simulink model "LKAS_AutoSave_20220216_1647"  (R2018b)
settings: Solver=FixedStepDiscrete  StartTime=0.0  StopTime=10.0  FixedStep=0.01  RelTol=1e-3
InitFcn:
  | tmpVer = ver('MATLAB');
  | tmpVer = str2num(tmpVer.Version);
  | % -------------------------------------------------------------------
  | %  MATLAB file generated by Simulink.saveVars on 21-Nov-2019 10:06:14
  | %  MATLAB version: 7.13.0.564 (R2011b)
  | % -------------------------------------------------------------------
  | 
  | 
  | SInt16 = Simulink.AliasType;
  | SInt16.Description = 'Num';
  | if (tmpVer > 7.11)
  | 	SInt16.DataScope = 'Auto';
  | end
  | SInt16.HeaderFile = 'Rte_Type.h';
  | SInt16.BaseType = 'int16';
  | 
  | SInt32 = Simulink.AliasType;
  | SInt32.Description = 'Num';
  | if (tmpVer > 7.11)
  | 	SInt32.DataScope = 'Auto';
  | end
  | SInt32.HeaderFile = 'Rte_Type.h';
  | SInt32.BaseType = 'int32';
  | 
  | SInt8 = Simulink.AliasType;
  | SInt8.Description = 'Num';
  | if (tmpVer > 7.11)
  | 	SInt8.DataScope = 'Auto';
  | end
  | SInt8.HeaderFile = 'Rte_Type.h';
  | SInt8.BaseType = 'int8';
  | 
  | T_A_m2_1024_1_u32 = Simulink.NumericType;
  | T_A_m2_1024_1_u32.Description = 'm2 (square meters  (m2))';
  | if (tmpVer > 7.11)
  | 	T_A_m2_1024_1_u32.DataScope = 'Auto';
  | end
  | T_A_m2_1024_1_u32.HeaderFile = 'Rte_Type.h';
  | T_A_m2_1024_1_u32.DataTypeMode = 'Fixed-point: slope and bias scaling';
  | T_A_m2_1024_1_u32.SignednessBool = false;
  | T_A_m2_1024_1_u32.WordLength = 32;
  | T_A_m2_1024_1_u32.FixedExponent = -10;
  | T_A_m2_1024_1_u32.SlopeAdjustmentFactor = 1;
  | T_A_m2_1024_1_u32.Bias = 0;
  | T_A_m2_1024_1_u32.DataTypeOverride = 'Inherit';
  | T_A_m2_1024_1_u32.IsAlias = true;
  | 
  | T_A_m2_65536_1_u16 = Simulink.NumericType;
  | T_A_m2_65536_1_u16.Description = 'm2 (square meters  (m2))';
  | if (tmpVer > 7.11)
  | 	T_A_m2_65536_1_u16.DataScope = 'Auto';
  | end
  | T_A_m2_65536_1_u16.HeaderFile = 'Rte_Type.h';
  | T_A_m2_65536_1_u16.DataTypeMode = 'Fixed-point: slope and bias scaling';
  | T_A_m2_65536_1_u16.SignednessBool = false;
  | T_A_m2_65536_1_u16.WordLength = 16;
  | T_A_m2_65536_1_u16.FixedExponent = -16;
  | T_A_m2_65536_1_u16.SlopeAdjustmentFactor = 1;
  | T_A_m2_65536_1_u16.Bias = 0;
  | T_A_m2_65536_1_u16.DataTypeOverride = 'Inherit';
  | ... (+4647 lines)
StopFcn:
  | clear  T_A_m2_1024_1_u32 T_A_m2_65536_1_u16 T_A_m2_Float32 T_A_mm2_10_1_u16 T_A_mm2_4_1_s16 T_A_mm2_Float32 T_Cnt_Num_10_1_u32 T_Cnt_Num_1_1_s16 T_Cnt_Num_1_1_s32 T_Cnt_Num_1_1_s8 T_Cnt_Num_1_1_u16 T_Cnt_Num_1_1_u32 T_Cnt_Num_1_1_u8 T_E_J_1_1_s32 T_E_J_Float32 T_E_kJ_128_1_s32 T_E_kJ_Float32 T_E_kwh_10_1_u16 T_E_kwh_Float32 T_Epl_kwhpkm_100_1_u16 T_Epl_kwhpkm_Float32 T_F_N_1_1_s16 T_F_N_Float32 T_I_A_1000_1_u16 T_I_A_1048576_1_s32 T_I_A_2048_1_s16 T_I_A_32_1_s16 T_I_A_Float32 T_I_mA_1_1_s16 T_I_mA_32768_128_s16 T_I_mA_Float32 T_J_kgpm2_128_1_u16 T_J_kgpm2_Float32 T_K_NA_1000_1_s16 T_K_NA_100_1_s16 T_K_NA_100_1_u16 T_K_NA_1024_1_s16 T_K_NA_1024_1_u16 T_K_NA_128_1_s16 T_K_NA_128_1_u16 T_K_NA_128_1_u8 T_K_NA_16777216_1_u32 T_K_NA_16_1_s16 T_K_NA_16_1_u16 T_K_NA_16_1_u8 T_K_NA_1_16_u16 T_K_NA_1_1_s16 T_K_NA_1_1_u16 T_K_NA_1_1_u8 T_K_NA_32768_1_s16 T_K_NA_32768_1_u16 T_K_NA_32_1_s8 T_K_NA_4096_1_u16 T_K_NA_4194304_1_s32 T_K_NA_4194304_1_u16 T_K_NA_65536_1_s32 T_K_NA_65536_1_u16 T_K_NA_8192_1_s16 T_K_NA_8_1_s16 T_K_NA_Float32 T_M_Nm_16_1_s16 T_M_Nm_1_1_s16 T_M_Nm_32768_1_s16 T_M_Nm_32_1_s16 T_M_Nm_4_1_s16 T_M_Nm_512_1_s16 T_M_Nm_Float32 T_P_W_1_4_s16 T_P_W_1_8_s16 T_P_W_Float32 T_P_kW_128_1_s16 T_P_kW_1_8_s16 T_P_kW_8_1_s32 T_P_kW_Float32 T_Pct_pct_1024_1_s32 T_Pct_pct_1024_1_u32 T_Pct_pct_10_1_s16 T_Pct_pct_10_1_u32 T_Pct_pct_128_100_s8 T_Pct_pct_1_1_s16 T_Pct_pct_1_4_u8 T_Pct_pct_255_100_u16 T_Pct_pct_255_100_u8 T_Pct_pct_256_1_s16 T_Pct_pct_256_1_u16 T_Pct_pct_65535_100_u16 T_Pct_pct_Float32 T_R_ohm_1024_1_s16 T_R_ohm_32_1_s16 T_R_ohm_Float32 T_TK_K_16_1_s16 T_TK_K_Float32 T_T_degC_10_400_1_u16 T_T_degC_16_1_s16 T_T_degC_1_40_1_u8 T_T_degC_2_80_1_u8 T_T_degC_Float32 T_U_V_1000_1_u16 T_U_V_10_1_u8 T_U_V_200_1_u8 T_U_V_32_1_s16 T_U_V_4096_1_s16 T_U_V_512_1_s16 T_U_V_65535_8_u16 T_U_V_8192_1_u16 T_U_V_Float32 T_U_mV_1_1_s16 T_U_mV_256_20_u16 T_U_mV_Float32 T_V_l_256_1_s16 T_V_l_4096_1_s16 T_V_l_64_1_s16 T_V_l_65535_100_u16 T_V_l_Float32 T_V_ml_128_1_s16 T_V_ml_1_1_s16 T_V_ml_32768_1_s16 T_V_ml_Float32 T_V_ul_32_1_u16 T_V_ul_Float32 T_Vpl_clpkm_512_1_u16 T_Vpl_clpkm_Float32 T_a_kphps_16_1_s16 T_a_kphps_Float32 T_a_mps2_128_1_s16 T_a_mps2_Float32 T_c_MJpkg_256_1_s16 T_c_MJpkg_Float32 T_c_kJpgpK_1024_1_s16 T_c_kJpgpK_Float32 T_c_kJpkgpK_128_1_u16 T_c_kJpkgpK_Float32 T_chrg_Ah_1_1_s16 T_chrg_Ah_1_1_u16 T_chrg_Ah_1_1_u8 T_chrg_Ah_256_1_u16 T_chrg_Ah_4194304_1_s32 T_chrg_Ah_512_1_u16 T_chrg_Ah_8_1_u16 T_chrg_Ah_Float32 T_cmp_NA_100_1_s16 T_cmp_NA_128_1_s16 T_cmp_NA_16_1_s16 T_cmp_NA_32768_1_u16 T_cmp_NA_Float32 T_d2n_rpmps2_4_1_s16 T_d2n_rpmps2_Float32 T_dPct_pctps_16_1_s16 T_dPct_pctps_256_1_s16 T_dPct_pctps_Float32 T_dT_degCps_128_1_s16 T_dT_degCps_Float32 T_dV_lph_1_1_s16 T_dV_lph_Float32 T_dV_lpm_128_1_s16 T_dV_lpm_32_1_s16 T_dV_lpm_Float32 T_dV_lps_1024_1_u16 T_dV_lps_4_1_u16 T_dV_lps_Float32 T_dV_mlps_1024_1_s16 T_dV_mlps_Float32 T_d_BitField16 T_dm_gps_128_1_s16 T_dm_gps_128_1_u16 T_dm_gps_256_1_u16 T_dm_gps_Float32 T_dm_mgps_1_1_s16 T_dm_mgps_Float32 T_dn_rpmps_1_1_s16 T_dn_rpmps_2_1_s16 T_dn_rpmps_Float32 T_dp_Paps_1_1_s16 T_dp_Paps_Float32 T_dp_kPaps_1_1_s16 T_dp_kPaps_8_1_s16 T_dp_kPaps_Float32 T_dphi_degps_128_1_s16 T_dphi_degps_8_1_s16 T_dphi_degps_Float32 T_dr_ps_256_1_s16 T_dr_ps_Float32 T_drho_mgplps_1_2_s16 T_drho_mgplps_Float32 T_e_NA_1_1_u8 T_f_Hz_1_1_u16 T_f_Hz_1_1_u32 T_f_Hz_64_1_u16 T_f_Hz_8_1_s16 T_f_Hz_Float32 T_g_BitField32 T_l_km_16_1_s16 T_l_km_1_1_u16 T_l_km_1_1_u32 T_l_km_Float32 T_l_m_1024_1_s16 T_l_m_16_1_s16 T_l_m_1_1_u32 T_l_m_Float32 T_l_mm_16_1_s16 T_l_mm_1_1_u16 T_l_mm_4096_1_s16 T_l_mm_4_1_u8 T_l_mm_64_1_s16 T_l_mm_Float32 T_m_g_1_1_s16 T_m_g_2048_1_s16 T_m_g_32_1_u16 T_m_g_Float32 T_m_kg_1024_1_s16 T_m_kg_1_1_s16 T_m_kg_1_1_u32 T_m_kg_Float32 T_m_mg_128_1_s16 T_m_mg_32_1_s16 T_m_mg_Float32 T_n_rpm_1_1_s16 T_n_rpm_1_25_u8 T_n_rpm_256_50_u16 T_n_rpm_2_25_u8 T_n_rpm_4_1_u16 T_n_rpm_Float32 T_p_MPa_64_1_s16 T_p_MPa_Float32 T_p_Pa_1_1_s16 T_p_Pa_Float32 T_p_kPa_1_10_u16 T_p_kPa_1_1_s16 T_p_kPa_1_1_u8 T_p_kPa_256_1_u16 T_p_kPa_32_1_u16 T_p_kPa_64_1_s16 T_p_kPa_Float32 T_phi_deg_100_1_s16 T_phi_deg_1024_1_s16 T_phi_deg_128_1_s16 T_phi_deg_1_1_u8 T_phi_deg_256_1_s16 T_phi_deg_2_1_s8 T_phi_deg_32_1_s16 T_phi_deg_512_6_s32 T_phi_deg_Float32 T_phi_rad_2048_1_s16 T_phi_rad_Float32 T_r_NA_1024_1_s16 T_r_NA_1024_1_u16 T_r_NA_16384_1_s16 T_r_NA_16_1_s16 T_r_NA_256_1_s8 T_r_NA_256_1_u16 T_r_NA_32768_1_u16 T_r_NA_32_1_u16 T_r_NA_4096_1_s16 T_r_NA_65535_2_u16 T_r_NA_8192_1_u16 T_r_NA_Float32 T_rho_gpl_8192_1_s16 T_rho_gpl_Float32 T_rho_kgpm3_16_1_s16 T_rho_kgpm3_Float32 T_rho_mgpl_1_1_s16 T_rho_mgpl_64_1_s16 T_rho_mgpl_Float32 T_t_hour_1_1_s16 T_t_hour_Float32 T_t_m_1_1_u16 T_t_m_Float32 T_t_ms_1_1_s16 T_t_ms_1_1_u16 T_t_ms_1_1_u32 T_t_ms_4096_1_s16 T_t_ms_64_1_s16 T_t_ms_Float32 T_t_s_1000_1_s16 T_t_s_100_1_s16 T_t_s_10_1_s16 T_t_s_10_1_u16 T_t_s_1_1_s16 T_t_s_1_1_u16 T_t_s_1_1_u32 T_t_s_Float32 T_t_us_10_1_u32 T_t_us_1_1_s16 T_t_us_1_1_u32 T_t_us_1_4_u16 T_t_us_Float32 T_v_kph_1_1_u8 T_v_kph_64_1_s16 T_v_kph_64_1_u16 T_v_kph_Float32 T_v_mps_256_1_s16 T_v_mps_Float32 T_w_radps_32_1_s16 T_w_radps_Float32 T_y_BitField8 T_y_BitFieldDiagProgress T_y_BitFieldDiagStatus T_y_NA_1_1_u8 SInt16 SInt32 SInt8 T_BOOLEAN UInt16 UInt32 UInt8 s16 s32 s8 u16 u32 u8
model workspace (MAT data in the model file):
  MCOS : class17 (value not decoded)
  MCOS : class17 (value not decoded)
  MCOS : class17 (value not decoded)
  MCOS : class17 (value not decoded)
  MCOS : class17 (value not decoded)
  MCOS : class17 (value not decoded)
  MCOS : class17 (value not decoded)
  MCOS : class17 (value not decoded)
  MCOS : class17 (value not decoded)
  MCOS : class17 (value not decoded)
  MCOS : class17 (value not decoded)
  MCOS : class17 (value not decoded)
  MCOS : class17 (value not decoded)
  MCOS : class17 (value not decoded)
  MCOS : class17 (value not decoded)
  MCOS : class17 (value not decoded)
  MCOS : class17 (value not decoded)
  MCOS : class17 (value not decoded)
  MCOS : class17 (value not decoded)
  MCOS : class17 (value not decoded)
  MCOS : class17 (value not decoded)
  MCOS : class17 (value not decoded)
  MCOS : class17 (value not decoded)
  MCOS : class17 (value not decoded)
  MCOS : class17 (value not decoded)
  MCOS : class17 (value not decoded)
  MCOS : class17 (value not decoded)
  MCOS : class17 (value not decoded)
  MCOS : class17 (value not decoded)
  MCOS : class17 (value not decoded)
  MCOS : class17 (value not decoded)
  MCOS : class17 (value not decoded)
  MCOS : class17 (value not decoded)
  MCOS : class17 (value not decoded)
  MCOS : class17 (value not decoded)
  MCOS : class17 (value not decoded)
  MCOS : class17 (value not decoded)
  MCOS : class17 (value not decoded)
  MCOS : class17 (value not decoded)
  MCOS : class17 (value not decoded)
  MCOS : class17 (value not decoded)
  MCOS : class17 (value not decoded)
  MCOS : class17 (value not decoded)
  MCOS : class17 (value not decoded)
  MCOS : class17 (value not decoded)
  MCOS : class17 (value not decoded)
  MCOS : class17 (value not decoded)
  MCOS : class17 (value not decoded)
  MCOS : class17 (value not decoded)
  MCOS : class17 (value not decoded)
  MCOS : class17 (value not decoded)
  MCOS : class17 (value not decoded)
  MCOS : class17 (value not decoded)
  MCOS : class17 (value not decoded)
  MCOS : class17 (value not decoded)
  MCOS : class17 (value not decoded)
  MCOS : class17 (value not decoded)
  MCOS : class17 (value not decoded)
  MCOS : class17 (value not decoded)
  MCOS : class17 (value not decoded)
  MCOS : class17 (value not decoded)
  MCOS : class17 (value not decoded)
  MCOS : class17 (value not decoded)
  MCOS : class17 (value not decoded)
  MCOS : class17 (value not decoded)
  MCOS : class17 (value not decoded)
  MCOS : class17 (value not decoded)
  MCOS : class17 (value not decoded)
  MCOS : class17 (value not decoded)
  MCOS : class17 (value not decoded)
  MCOS : class17 (value not decoded)
  MCOS : class17 (value not decoded)
  MCOS : class17 (value not decoded)
  MCOS : class17 (value not decoded)
  MCOS : class17 (value not decoded)
  MCOS : class17 (value not decoded)
  MCOS : class17 (value not decoded)
  MCOS : class17 (value not decoded)
  MCOS : class17 (value not decoded)
  MCOS : class17 (value not decoded)
  MCOS : class17 (value not decoded)
  MCOS : class17 (value not decoded)
  MCOS : class17 (value not decoded)
  MCOS : class17 (value not decoded)
  MCOS : class17 (value not decoded)
  MCOS : class17 (value not decoded)
  MCOS : class17 (value not decoded)
  MCOS : class17 (value not decoded)
  MCOS : class17 (value not decoded)
  MCOS : class17 (value not decoded)
  MCOS : class17 (value not decoded)
  MCOS : class17 (value not decoded)
  MCOS : class17 (value not decoded)
  MCOS : class17 (value not decoded)
  MCOS : class17 (value not decoded)
  MCOS : class17 (value not decoded)
  MCOS : class17 (value not decoded)
  MCOS : class17 (value not decoded)
  MCOS : class17 (value not decoded)
  MCOS : class17 (value not decoded)
  MCOS : class17 (value not decoded)
  MCOS : class17 (value not decoded)
undefined symbols (not defined in the file): LKA_CarWidth, LKA_SampleTime, LKA_StrRatio_C, LKA_Veh2CamL_C, LKA_Veh2CamW_C, LKA_WhlBaseL_C, LL_CompHdAg_C, LL_CompSWA_C, LL_CrvtPrvwT_C, LL_DesDvt_C, LL_DvtComp_C, LL_DvtPrvwT_C, LL_DvtSpdDet_vDvtSpdMin_C, LL_HandsOff_ExitTime, LL_HandsOff_TextTime, LL_HandsOff_WarnTime, LL_HdAgExT_C, LL_HdAgPrvwT_C, LL_LAccMax_C, LL_LAccRMax_C, LL_LDW_EarliestWarnLine_C, LL_LDW_LatestWarnLine_C, LL_LDWS_SUPPRESS_HEADING, LL_LFClb_TFC_FfCtlRatio_C, LL_LFClb_TFC_KdBalance_C, LL_LFClb_TFC_KdMaxSWA_C, LL_LFClb_TFC_KdV1_C, LL_LFClb_TFC_KdV2_C, LL_LFClb_TFC_KdVehSpdLwr_C, LL_LFClb_TFC_KdVehSpdUpr_C, LL_LFClb_TFC_Ki_C, LL_LFClb_TFC_KiMaxSWA_C, LL_LFClb_TFC_Kp_C, LL_LFClb_TFC_KpKlat_C, LL_LFClb_TFC_KpV1_C, LL_LFClb_TFC_KpV2_C, LL_LFClb_TFC_KpVehSpdLwr_C, LL_LFClb_TFC_KpVehSpdUpr_C, LL_LFClb_TFC_PrvwT_C, LL_LKA_EarliestWarnLine_C, LL_LKA_LatestWarnLine_C, LL_LKAExPrcs_ExitC0Dvt, LL_LKAExPrcs_ExitC0Swt, LL_LKAExPrcs_tiExitTime1, LL_LKAExPrcs_tiExitTime2, LL_LKAExPrcs_tiExitTime3, LL_LKAS_OUT_OF_CONTROL_LAT_VEL, LL_LKAS_OUT_OF_CONTROL_TTLC, LL_LKASWASyn_M0, LL_LKASWASyn_M1, LL_LKASWASyn_M2, LL_LKASWASyn_M3K, LL_LKASWASyn_SWAaddMax, LL_LKASWASyn_T2, LL_LKASWASyn_tiTrqSwaRtTime, LL_LKASWASyn_tiTrqSwaTime, LL_LKASWASyn_TrqMax, LL_LKASWASyn_TrqSwaAddSwt, LL_LKASWASyn_TrqSwaRateDiff, LL_LSpdCompT_C ... (+43)
libraries: simulink x136, canmsglib x8, dspstat3 x3, simulink_extras x1
(part 16 of 20)

== system LKAS_AutoSave_20220216_1647/LKAS/LL/LLOn/LL State Determination (LLStateDet)/LL State Machine Conditions (LLSMCon)/Disable Condition (DisblC)/Driver Intent Condition (DrvInttC)/Driver Action Detection (DrvActnDet) ==
  DrvActnDet_phiSWA : Inport
  DrvActnDet_dphiSWA_Speed : Inport  Port=2
  DrvActnDet_aLAcc : Inport  Port=3
  DrvActnDet_aFAcc : Inport  Port=4
  DrvActnDet_bsEPSInfo : Inport  Port=5
  DrvInttC_bsLLClb : Inport  Port=6
  Abs2 : Abs  OutDataTypeStr=single
  Abs3 : Abs  OutDataTypeStr=single
  Abs4 : Abs  OutDataTypeStr=single
  Bus Creator : BusCreator  Inputs=4
  Bus Selector : BusSelector  OutputSignals=EPS_LKA_State
  Bus Selector1 : BusSelector  OutputSignals=bsLLSMConClb.DisblCClb.LL_MAX_STEER_ANGLE_DISABLE,bsLLSMConClb.DisblCClb.LL_MAX_STEER_SPEED_DISABLE,bsLLSMConClb.DisblCClb.LL_MAX_LAT_ACC_DISABLE,bsLLSMConClb.DisblCClb.LL_MAX_LONG_ACC_DISABLE,bsLLSMConClb.DisblCClb.LL_MAX_LONG_DECEL_DISABLE
  Compare To Constant : simulink/Logic and Bit Operations/Compare To Constant  relop=~=  const=3.0  OutDataTypeStr=boolean
  Compare To Constant2 : simulink/Logic and Bit Operations/Compare To Constant  relop===  const=0  OutDataTypeStr=boolean
  Interval Test Dynamic : simulink/Logic and Bit Operations/Interval Test Dynamic  IntervalClosedRight=off  IntervalClosedLeft=off  OutDataTypeStr=boolean
      settings: SourceProductName=Simulink  SourceProductBaseCode=SL
  Logical Operator : Logic  Operator=OR  Inputs=4  AllPortsSameDT=off  OutDataTypeStr=boolean
  Logical Operator1 : Logic  AllPortsSameDT=off  OutDataTypeStr=boolean
  Relational Operator1 : RelationalOperator  OutDataTypeStr=boolean  RndMeth=Nearest
  Relational Operator2 : RelationalOperator  OutDataTypeStr=boolean  RndMeth=Nearest
  Relational Operator3 : RelationalOperator  OutDataTypeStr=boolean  RndMeth=Nearest
  Unary Minus : UnaryMinus
  DrvActnDet_stTkOvStActvFlg : Outport
  DrvActnDet : Outport  Port=2
  wires:
  Abs2/1 -> Relational Operator1/1
  Bus Selector1/1 -> Relational Operator1/2  "<LL_MAX_STEER_ANGLE_DISABLE>"
  Abs3/1 -> Relational Operator2/1
  Bus Selector1/2 -> Relational Operator2/2  "<LL_MAX_STEER_SPEED_DISABLE>"
  DrvActnDet_phiSWA/1 -> Abs2/1
  DrvActnDet_aLAcc/1 -> Abs4/1
  Abs4/1 -> Relational Operator3/1
  Bus Selector1/3 -> Relational Operator3/2  "<LL_MAX_LAT_ACC_DISABLE>"
  Bus Selector1/5 -> Unary Minus/1  "<LL_MAX_LONG_DECEL_DISABLE>"
  DrvActnDet_aFAcc/1 -> Interval Test Dynamic/2
  Interval Test Dynamic/1 -> Compare To Constant2/1
  Bus Selector1/4 -> Interval Test Dynamic/1  "<LL_MAX_LONG_ACC_DISABLE>"
  Unary Minus/1 -> Interval Test Dynamic/3
  Relational Operator3/1 -> Logical Operator1/1
  DrvActnDet_bsEPSInfo/1 -> Bus Selector/1
  Bus Selector/1 -> Compare To Constant/1  "<EPS_LKA_State>"
  Compare To Constant/1 -> Logical Operator1/2
  Logical Operator/1 -> DrvActnDet_stTkOvStActvFlg/1
  Relational Operator1/1 -> Bus Creator/1, Logical Operator/1  "phiSWA_Thres"
  Bus Creator/1 -> DrvActnDet/1
  Compare To Constant2/1 -> Bus Creator/4, Logical Operator/4  "aFLAcc_Thres"
  Logical Operator1/1 -> Bus Creator/3, Logical Operator/3  "aLAcc_Thres"
  Relational Operator2/1 -> Bus Creator/2, Logical Operator/2  "dphiSWARate_Thres"
  DrvActnDet_dphiSWA_Speed/1 -> Abs3/1
  DrvInttC_bsLLClb/1 -> Bus Selector1/1

== system LKAS_AutoSave_20220216_1647/LKAS/LL/LLOn/LL State Determination (LLStateDet)/LL State Machine Conditions (LLSMCon)/Disable Condition (DisblC)/Driver Intent Condition (DrvInttC)/Driver Release Detection (DrvRlsDet) ==
  DrvRlsDet_bsEPSInfo : Inport
  DrvRlsDet_bsLLClb : Inport  Port=2
  Abs : Abs
  Bus Selector2 : BusSelector  OutputSignals=EPS_LKA_State,EPS_SW_Trq
  Bus Selector3 : BusSelector  OutputSignals=bsLLSMConClb.DisblCClb.LL_RlsDet_tiTrqChkT_DISABLE,bsLLSMConClb.DisblCClb.LL_RlsDet_tiTrqChkT_EPS_DISABLE,bsConstantClb.LKA_SampleTime,bsLLSMConClb.DisblCClb.LL_HandsOff_ExitTime
  Compare1 : simulink/Logic and Bit Operations/Compare To Constant  relop===  const=3  OutDataTypeStr=boolean
  Compare3 : simulink/Logic and Bit Operations/Compare To Constant  relop===  const=3  OutDataTypeStr=boolean
  Compare4 : simulink/Logic and Bit Operations/Compare To Constant  relop===  const=1  OutDataTypeStr=boolean
  Divide : Product  Inputs=**
  ExitCount : Subsystem
  Logical Operator1 : Logic  AllPortsSameDT=off  OutDataTypeStr=boolean
  Logical Operator2 : Logic  Operator=OR  AllPortsSameDT=off  OutDataTypeStr=boolean
  Relational Operator : RelationalOperator  Operator=<=  OutDataTypeStr=boolean  RndMeth=Nearest
  Switch : Switch  Criteria=u2 > Threshold
  DrvRlsDet_stDrvRlsDetFlg : Outport
  wires:
  Logical Operator1/1 -> Divide/1
  DrvRlsDet_bsEPSInfo/1 -> Bus Selector2/1
  Bus Selector2/1 -> Compare1/1, Compare4/1, Compare3/1  "<EPS_LKA_State>"
  Bus Selector2/2 -> Abs/1  "<EPS_SW_Trq>"
  Relational Operator/1 -> ExitCount/Enable, Logical Operator1/2
  Compare1/1 -> Switch/2
  Compare3/1 -> Logical Operator2/2
  Bus Selector3/2 -> Switch/1  "<LL_RlsDet_tiTrqChkT_EPS_DISABLE>"
  Switch/1 -> Relational Operator/2
  Logical Operator2/1 -> Logical Operator1/1
  Compare4/1 -> Logical Operator2/1
  Abs/1 -> Relational Operator/1
  DrvRlsDet_bsLLClb/1 -> Bus Selector3/1
  Bus Selector3/1 -> Switch/3  "<LL_RlsDet_tiTrqChkT_DISABLE>"
  Bus Selector3/3 -> Divide/2  "<LKA_SampleTime>"
  Bus Selector3/4 -> ExitCount/2(ExitTime)  "<LL_HandsOff_ExitTime>"
  ExitCount/1(Out) -> DrvRlsDet_stDrvRlsDetFlg/1
  Divide/1 -> ExitCount/1(SampleTime)

== system LKAS_AutoSave_20220216_1647/LKAS/LL/LLOn/LL State Determination (LLStateDet)/LL State Machine Conditions (LLSMCon)/Disable Condition (DisblC)/Driver Intent Condition (DrvInttC)/Take-Over Steering Check (TkOvStChk) ==
  TkOvStChk_bsEPSInfo : Inport
  TkOvStChk_bsLLClb : Inport  Port=2
  TkOvStChk_bsVehSpd : Inport  Port=3
  TkOvStChk_crPrvwCrvt : Inport  Port=4
  Abs : Abs
  Bus Selector : BusSelector  OutputSignals=EPS_SW_Trq
  Bus Selector1 : BusSelector  OutputSignals=bsLLSMConClb.DisblCClb.LL_MAX_DRIVER_TORQUE_DISABLE,bsLLSMConClb.DisblCClb.LL_TkOvStChk_tiTrqChkT,bsLLSMConClb.DisblCClb.LL_TkOvStChk_tiTDelTime,bsConstantClb.LKA_SampleTime
  MATLAB Function : MATLAB Function  TreatAsAtomicUnit=on
  Saturation : Saturate  UpperLimit=80  LowerLimit=60
      settings: AttributesFormatString="Min = %<LowerLimit>  Max = %<UpperLimit>"
  Sum Condition1 : Subsystem  TreatAsAtomicUnit=on
  Time Delay (TDel) : Subsystem
  TkOvStChk_stTkOvStChk : Outport
  wires:
  Sum Condition1/1(Out) -> Time Delay (TDel)/1(TDel_stFlgIn)
  Saturation/1 -> MATLAB Function/1(VehSpd)
  TkOvStChk_bsEPSInfo/1 -> Bus Selector/1
  Bus Selector/1 -> Abs/1  "<EPS_SW_Trq>"
  Abs/1 -> MATLAB Function/2(EPSTrq)
  Bus Selector1/1 -> MATLAB Function/3(DisableTrq)  "<LL_MAX_DRIVER_TORQUE_DISABLE>"
  MATLAB Function/1(stDvrTkConFlg) -> Sum Condition1/Enable
  Bus Selector1/2 -> Sum Condition1/2(Sum)  "<LL_TkOvStChk_tiTrqChkT>"
  Time Delay (TDel)/1(TDel_stFlgOut) -> TkOvStChk_stTkOvStChk/1
  TkOvStChk_bsVehSpd/1 -> Saturation/1
  Bus Selector1/3 -> Time Delay (TDel)/3(TDel_tiTDel)  "<LL_TkOvStChk_tiTDelTime>"
  Bus Selector1/4 -> Sum Condition1/1(In), Time Delay (TDel)/2(SampleTime)  "<LKA_SampleTime>"
  TkOvStChk_crPrvwCrvt/1 -> MATLAB Function/4(PrvwCrvt)
  TkOvStChk_bsLLClb/1 -> Bus Selector1/1

== system LKAS_AutoSave_20220216_1647/LKAS/LL/LLOn/LL State Determination (LLStateDet)/LL State Machine Conditions (LLSMCon)/Disable Condition (DisblC)/LDW Alarm Timeout (LDWAlrmTOut)/If Action Subsystem ==
  In : Inport
  Sum : Inport  Port=2
  Action Port : ActionPort  InitializeStates=reset
      settings: AttributesFormatString=states = %<InitializeStates>
  Add1 : Sum  OutDataTypeStr=single
  Memory : Memory  InheritSampleTime=on
  Relational Operator : RelationalOperator  OutDataTypeStr=boolean  RndMeth=Nearest
  Saturation : Saturate  UpperLimit=10  LowerLimit=0
      settings: AttributesFormatString="Min = %<LowerLimit>  Max = %<UpperLimit>"
  Out : Outport  InitialOutput=0
      settings: AttributesFormatString=%<OutputWhenDisabled> = %<InitialOutput>
  wires:
  Sum/1 -> Relational Operator/2
  In/1 -> Add1/1
  Memory/1 -> Add1/2
  Saturation/1 -> Memory/1, Relational Operator/1
  Add1/1 -> Saturation/1
  Relational Operator/1 -> Out/1

== system LKAS_AutoSave_20220216_1647/LKAS/LL/LLOn/LL State Determination (LLStateDet)/LL State Machine Conditions (LLSMCon)/Disable Condition (DisblC)/LDW Alarm Timeout (LDWAlrmTOut)/If Action Subsystem1 ==
  Action Port : ActionPort  InitializeStates=reset
      settings: AttributesFormatString=states = %<InitializeStates>
  Constant : Constant  Value=0  OutDataTypeStr=boolean
  Out1 : Outport  InitialOutput=0
      settings: AttributesFormatString=%<OutputWhenDisabled> = %<InitialOutput>
  wires:
  Constant/1 -> Out1/1

== system LKAS_AutoSave_20220216_1647/LKAS/LL/LLOn/LL State Determination (LLStateDet)/LL State Machine Conditions (LLSMCon)/Disable Condition (DisblC)/LKA Own Condition (LKAOwnC)/EPS Condition (EPSC) ==
  EPSC_tiDelT_C : Inport
  EPSC_tiLKA_SampleTime : Inport  Port=2
  EPSC_bsEPSInfo : Inport  Port=3
  EPSC_bsLLState : Inport  Port=4
  Bus Selector : BusSelector  OutputSignals=EPS_LKA_State
  Bus Selector1 : BusSelector  OutputSignals=LKA_State
  If : If  NumInputs=2  IfExpression=u2 ==3 & u1 ~=1  ElseIfExpressions=(u2 == 4 | u2 == 5)& u1 ~= 3
  If Action Subsystem : Subsystem  TreatAsAtomicUnit=on
  If Action Subsystem1 : Subsystem  TreatAsAtomicUnit=on
  If Action Subsystem3 : Subsystem  TreatAsAtomicUnit=on
  Merge : Merge  Inputs=3
  Sum Condition1 : Subsystem  TreatAsAtomicUnit=on
  EPSC_stEPSC : Outport
  wires:
  EPSC_bsEPSInfo/1 -> Bus Selector/1
  Sum Condition1/1(Out) -> EPSC_stEPSC/1
  If Action Subsystem1/1(Out) -> Merge/2
  If Action Subsystem/1(Out) -> Merge/1
  If/1 -> If Action Subsystem/Action
  If/3 -> If Action Subsystem3/Action
  If/2 -> If Action Subsystem1/Action
  If Action Subsystem3/1(Out) -> Merge/3
  Merge/1 -> Sum Condition1/Enable
  Bus Selector/1 -> If/1  "<EPS_LKA_State>"
  EPSC_bsLLState/1 -> Bus Selector1/1
  Bus Selector1/1 -> If/2  "<LKA_State>"
  EPSC_tiDelT_C/1 -> Sum Condition1/2(Sum)
  EPSC_tiLKA_SampleTime/1 -> Sum Condition1/1(SampleTime)

== system LKAS_AutoSave_20220216_1647/LKAS/LL/LLOn/LL State Determination (LLStateDet)/LL State Machine Conditions (LLSMCon)/Disable Condition (DisblC)/LKA Own Condition (LKAOwnC)/LKA Own Condition Synthesis (LKAOwnCSyn) ==
  LKAOwnCSyn_stDACMode : Inport
  LKAOwnCSyn_stVehLSpdC : Inport  Port=2
  LKAOwnCSyn_stVehPosChk : Inport  Port=3
  LKAOwnCSyn_stEPSCtlEC : Inport  Port=4
  Compare To Constant : simulink/Logic and Bit Operations/Compare To Constant  relop===  const=2  OutDataTypeStr=boolean
  Compare To Constant1 : simulink/Logic and Bit Operations/Compare To Constant  relop===  const=1  OutDataTypeStr=boolean
  Compare To Constant2 : simulink/Logic and Bit Operations/Compare To Constant  relop===  const=1  OutDataTypeStr=boolean
  Compare To Constant3 : simulink/Logic and Bit Operations/Compare To Constant  relop===  const=1  OutDataTypeStr=boolean
  Logical Operator : Logic  AllPortsSameDT=off  OutDataTypeStr=boolean
  Logical Operator1 : Logic  Operator=OR  Inputs=3  AllPortsSameDT=off  OutDataTypeStr=boolean
  LKAOwnCSyn_stLKAOwnCSyn : Outport
  wires:
  LKAOwnCSyn_stDACMode/1 -> Compare To Constant/1
  LKAOwnCSyn_stVehPosChk/1 -> Compare To Constant1/1
  Logical Operator/1 -> LKAOwnCSyn_stLKAOwnCSyn/1
  LKAOwnCSyn_stEPSCtlEC/1 -> Compare To Constant2/1
  Compare To Constant2/1 -> ?
  Compare To Constant1/1 -> Logical Operator1/2
  Compare To Constant/1 -> Logical Operator/1
  Logical Operator1/1 -> Logical Operator/2
  LKAOwnCSyn_stVehLSpdC/1 -> Compare To Constant3/1
  Compare To Constant3/1 -> Logical Operator1/1

== system LKAS_AutoSave_20220216_1647/LKAS/LL/LLOn/LL State Determination (LLStateDet)/LL State Machine Conditions (LLSMCon)/Disable Condition (DisblC)/LKA Own Condition (LKAOwnC)/Vehicle Lateral Speed Condition (VehLSpdC) ==
  VehLSpdC_bsTTLC : Inport
  VehLSpdC_vVehLSpdMax_C : Inport  Port=2
  Abs : Abs
  Abs1 : Abs
  Bus Selector : BusSelector  OutputSignals=vLft,vRgt
  Logical Operator : Logic  Operator=OR  AllPortsSameDT=off  OutDataTypeStr=boolean
  Relational Operator1 : RelationalOperator  OutDataTypeStr=boolean  RndMeth=Nearest
  Relational Operator2 : RelationalOperator  OutDataTypeStr=boolean  RndMeth=Nearest
  VehLSpdC_stVehLSpdC : Outport
  wires:
  VehLSpdC_bsTTLC/1 -> Bus Selector/1
  Abs/1 -> Relational Operator1/1
  Bus Selector/1 -> Abs/1  "<vLft>"
  Bus Selector/2 -> Abs1/1  "<vRgt>"
  Abs1/1 -> Relational Operator2/1
  VehLSpdC_vVehLSpdMax_C/1 -> Relational Operator2/2, Relational Operator1/2
  Relational Operator1/1 -> Logical Operator/1
  Relational Operator2/1 -> Logical Operator/2
  Logical Operator/1 -> VehLSpdC_stVehLSpdC/1

== system LKAS_AutoSave_20220216_1647/LKAS/LL/LLOn/LL State Determination (LLStateDet)/LL State Machine Conditions (LLSMCon)/Disable Condition (DisblC)/LKA Own Condition (LKAOwnC)/Vehicle Position Check (VehPosChk) ==
  VehPosChk_lLftDvt : Inport
  VehPosChk_lRgtDvt : Inport  Port=2
  VehPosChk_lAlrmLine_C : Inport  Port=3
  Logical Operator : Logic  Operator=OR  AllPortsSameDT=off  OutDataTypeStr=boolean
  Relational Operator1 : RelationalOperator  Operator=<=  OutDataTypeStr=boolean  RndMeth=Nearest
  Relational Operator2 : RelationalOperator  Operator=<=  OutDataTypeStr=boolean  RndMeth=Nearest
  VehPosChk_stVehPosChk : Outport
  wires:
  VehPosChk_lAlrmLine_C/1 -> Relational Operator1/2, Relational Operator2/2
  Relational Operator1/1 -> Logical Operator/1
  Relational Operator2/1 -> Logical Operator/2
  Logical Operator/1 -> VehPosChk_stVehPosChk/1
  VehPosChk_lLftDvt/1 -> Relational Operator1/1
  VehPosChk_lRgtDvt/1 -> Relational Operator2/1

== system LKAS_AutoSave_20220216_1647/LKAS/LL/LLOn/LL State Determination (LLStateDet)/LL State Machine Conditions (LLSMCon)/Disable Condition (DisblC)/Lane Condition (LaneC)/Lane C1 Detection (LaneC1Det) ==
  LaneWDet_facmL0C1 : Inport
  LaneWDet_facmR0C1 : Inport  Port=2
  Abs : Abs
  Add : Sum  Inputs=+-  OutDataTypeStr=single
  Compare To Constant1 : simulink/Logic and Bit Operations/Compare To Constant  relop=>  const=0.040  OutDataTypeStr=boolean
  LaneC1Det_stLaneC1DetFlg : Outport
  wires:
  LaneWDet_facmR0C1/1 -> Add/2
  LaneWDet_facmL0C1/1 -> Add/1
  Add/1 -> Abs/1
  Compare To Constant1/1 -> LaneC1Det_stLaneC1DetFlg/1
  Abs/1 -> Compare To Constant1/1

== system LKAS_AutoSave_20220216_1647/LKAS/LL/LLOn/LL State Determination (LLStateDet)/LL State Machine Conditions (LLSMCon)/Disable Condition (DisblC)/Lane Condition (LaneC)/Lane Condition Synthesis (LaneCSyn) ==
  LaneCSyn_stLaneQlECFlg : Inport
  LaneCSyn_stLaneWDetFlg : Inport  Port=2
  LaneCSyn_stLaneCrvtDetFlg : Inport  Port=3
  LaneCSyn_stLaneC1DetFlg : Inport  Port=4
  Logical Operator3 : Logic  Operator=OR  Inputs=4  AllPortsSameDT=off  OutDataTypeStr=boolean
  LaneCSyn_stLaneCSyn : Outport
  wires:
  LaneCSyn_stLaneQlECFlg/1 -> Logical Operator3/1
  LaneCSyn_stLaneCrvtDetFlg/1 -> Logical Operator3/3
  Logical Operator3/1 -> LaneCSyn_stLaneCSyn/1
  LaneCSyn_stLaneWDetFlg/1 -> Logical Operator3/2
  LaneCSyn_stLaneC1DetFlg/1 -> Logical Operator3/4

== system LKAS_AutoSave_20220216_1647/LKAS/LL/LLOn/LL State Determination (LLStateDet)/LL State Machine Conditions (LLSMCon)/Disable Condition (DisblC)/Lane Condition (LaneC)/Lane Curvature Detection (LaneCrvtDet) ==
  LaneCrvtDet_crPrvwCrvt : Inport
  LaneCrvtDet_crLaneCrvtMax_C : Inport  Port=2
  Abs : Abs
  Constant : Constant  Value=0  OutDataTypeStr=single  SampleTime=-1
  Interval Test Dynamic : simulink/Logic and Bit Operations/Interval Test Dynamic  IntervalClosedRight=on  IntervalClosedLeft=on  OutDataTypeStr=boolean
      settings: SourceProductName=Simulink  SourceProductBaseCode=SL
  Logical Operator : Logic  Operator=NOT  AllPortsSameDT=off  OutDataTypeStr=boolean
  LaneCrvtDet_stLaneCrvtDetFlg : Outport
  wires:
  Interval Test Dynamic/1 -> Logical Operator/1
  Logical Operator/1 -> LaneCrvtDet_stLaneCrvtDetFlg/1
  LaneCrvtDet_crLaneCrvtMax_C/1 -> Interval Test Dynamic/1
  Constant/1 -> Interval Test Dynamic/3
  LaneCrvtDet_crPrvwCrvt/1 -> Abs/1
  Abs/1 -> Interval Test Dynamic/2

== system LKAS_AutoSave_20220216_1647/LKAS/LL/LLOn/LL State Determination (LLStateDet)/LL State Machine Conditions (LLSMCon)/Disable Condition (DisblC)/Lane Condition (LaneC)/Lane Quality Disable Condition (LaneQlDC) ==
  LaneQlDC_stFacmL0Ql : Inport
  LaneQlDC_stFacmR0Ql : Inport  Port=2
  Compare To Constant : simulink/Logic and Bit Operations/Compare To Constant  relop=<  const=3  OutDataTypeStr=boolean
  Compare To Constant1 : simulink/Logic and Bit Operations/Compare To Constant  relop=<  const=3  OutDataTypeStr=boolean
  Logical Operator : Logic  AllPortsSameDT=off  OutDataTypeStr=boolean
  LaneQlDC_stLaneQlDCFlg : Outport
  wires:
  LaneQlDC_stFacmL0Ql/1 -> Compare To Constant/1
  LaneQlDC_stFacmR0Ql/1 -> Compare To Constant1/1
  Compare To Constant/1 -> Logical Operator/1
  Compare To Constant1/1 -> Logical Operator/2
  Logical Operator/1 -> LaneQlDC_stLaneQlDCFlg/1

== system LKAS_AutoSave_20220216_1647/LKAS/LL/LLOn/LL State Determination (LLStateDet)/LL State Machine Conditions (LLSMCon)/Disable Condition (DisblC)/Lane Condition (LaneC)/Lane Width Detection (LaneWDet) ==
  LaneWDet_LaneWidth : Inport
  LaneWDet_lLaneWMax : Inport  Port=2
  LaneWDet_lLaneWMin : Inport  Port=3
  Abs1 : Abs
  Compare To Zero : simulink/Logic and Bit Operations/Compare To Zero  relop===  OutDataTypeStr=boolean
  Interval Test Dynamic : simulink/Logic and Bit Operations/Interval Test Dynamic  IntervalClosedRight=on  IntervalClosedLeft=on  OutDataTypeStr=boolean
      settings: SourceProductName=Simulink  SourceProductBaseCode=SL
  LaneWDet_stLaneWDetFlg : Outport
  wires:
  Interval Test Dynamic/1 -> Compare To Zero/1
  Compare To Zero/1 -> LaneWDet_stLaneWDetFlg/1
  LaneWDet_lLaneWMax/1 -> Interval Test Dynamic/1
  LaneWDet_lLaneWMin/1 -> Interval Test Dynamic/3
  Abs1/1 -> Interval Test Dynamic/2
  LaneWDet_LaneWidth/1 -> Abs1/1

== system LKAS_AutoSave_20220216_1647/LKAS/LL/LLOn/LL State Determination (LLStateDet)/LL State Machine Conditions (LLSMCon)/Disable Condition (DisblC)/Subsystem/Subsystem ==
  in1 : Inport
  Add : Sum
  Cast To Single : DataTypeConversion  OutDataTypeStr=uint8
  Memory : Memory  InheritSampleTime=on
  Saturation : Saturate  UpperLimit=1  LowerLimit=0
      settings: AttributesFormatString="Min = %<LowerLimit>  Max = %<UpperLimit>"
  Out1 : Outport
  wires:
  Cast To Single/1 -> Add/1
  in1/1 -> Cast To Single/1
  Memory/1 -> Saturation/1
  Add/1 -> Memory/1
  Saturation/1 -> Add/2, Out1/1

== system LKAS_AutoSave_20220216_1647/LKAS/LL/LLOn/LL State Determination (LLStateDet)/LL State Machine Conditions (LLSMCon)/Disable Condition (DisblC)/Subsystem/Subsystem1 ==
  in1 : Inport
  Add : Sum
  Cast To Single : DataTypeConversion  OutDataTypeStr=uint8
  Memory : Memory  InheritSampleTime=on
  Saturation : Saturate  UpperLimit=1  LowerLimit=0
      settings: AttributesFormatString="Min = %<LowerLimit>  Max = %<UpperLimit>"
  Out1 : Outport
  wires:
  Saturation/1 -> Out1/1, Add/2
  Add/1 -> Memory/1
  Memory/1 -> Saturation/1
  in1/1 -> Cast To Single/1
  Cast To Single/1 -> Add/1

== system LKAS_AutoSave_20220216_1647/LKAS/LL/LLOn/LL State Determination (LLStateDet)/LL State Machine Conditions (LLSMCon)/Disable Condition (DisblC)/Subsystem/Subsystem10 ==
  in1 : Inport
  Add : Sum
  Cast To Single : DataTypeConversion  OutDataTypeStr=uint8
  Memory : Memory  InheritSampleTime=on
  Saturation : Saturate  UpperLimit=1  LowerLimit=0
      settings: AttributesFormatString="Min = %<LowerLimit>  Max = %<UpperLimit>"
  Out1 : Outport
  wires:
  Cast To Single/1 -> Add/1
  in1/1 -> Cast To Single/1
  Memory/1 -> Saturation/1
  Add/1 -> Memory/1
  Saturation/1 -> Add/2, Out1/1

== system LKAS_AutoSave_20220216_1647/LKAS/LL/LLOn/LL State Determination (LLStateDet)/LL State Machine Conditions (LLSMCon)/Disable Condition (DisblC)/Subsystem/Subsystem11 ==
  in1 : Inport
  Add : Sum
  Cast To Single : DataTypeConversion  OutDataTypeStr=uint8
  Memory : Memory  InheritSampleTime=on
  Saturation : Saturate  UpperLimit=1  LowerLimit=0
      settings: AttributesFormatString="Min = %<LowerLimit>  Max = %<UpperLimit>"
  Out1 : Outport
  wires:
  Saturation/1 -> Out1/1, Add/2
  Add/1 -> Memory/1
  Memory/1 -> Saturation/1
  in1/1 -> Cast To Single/1
  Cast To Single/1 -> Add/1

== system LKAS_AutoSave_20220216_1647/LKAS/LL/LLOn/LL State Determination (LLStateDet)/LL State Machine Conditions (LLSMCon)/Disable Condition (DisblC)/Subsystem/Subsystem12 ==
  in1 : Inport
  Add : Sum
  Cast To Single : DataTypeConversion  OutDataTypeStr=uint8
  Memory : Memory  InheritSampleTime=on
  Saturation : Saturate  UpperLimit=1  LowerLimit=0
      settings: AttributesFormatString="Min = %<LowerLimit>  Max = %<UpperLimit>"
  Out1 : Outport
  wires:
  Cast To Single/1 -> Add/1
  in1/1 -> Cast To Single/1
  Memory/1 -> Saturation/1
  Add/1 -> Memory/1
  Saturation/1 -> Add/2, Out1/1

== system LKAS_AutoSave_20220216_1647/LKAS/LL/LLOn/LL State Determination (LLStateDet)/LL State Machine Conditions (LLSMCon)/Disable Condition (DisblC)/Subsystem/Subsystem13 ==
  in1 : Inport
  Add : Sum
  Cast To Single : DataTypeConversion  OutDataTypeStr=uint8
  Memory : Memory  InheritSampleTime=on
  Saturation : Saturate  UpperLimit=1  LowerLimit=0
      settings: AttributesFormatString="Min = %<LowerLimit>  Max = %<UpperLimit>"
  Out1 : Outport
  wires:
  Saturation/1 -> Out1/1, Add/2
  Add/1 -> Memory/1
  Memory/1 -> Saturation/1
  in1/1 -> Cast To Single/1
  Cast To Single/1 -> Add/1

== system LKAS_AutoSave_20220216_1647/LKAS/LL/LLOn/LL State Determination (LLStateDet)/LL State Machine Conditions (LLSMCon)/Disable Condition (DisblC)/Subsystem/Subsystem14 ==
  in1 : Inport
  Add : Sum
  Cast To Single : DataTypeConversion  OutDataTypeStr=uint8
  Memory : Memory  InheritSampleTime=on
  Saturation : Saturate  UpperLimit=1  LowerLimit=0
      settings: AttributesFormatString="Min = %<LowerLimit>  Max = %<UpperLimit>"
  Out1 : Outport
  wires:
  Saturation/1 -> Out1/1, Add/2
  Add/1 -> Memory/1
  Memory/1 -> Saturation/1
  in1/1 -> Cast To Single/1
  Cast To Single/1 -> Add/1

== system LKAS_AutoSave_20220216_1647/LKAS/LL/LLOn/LL State Determination (LLStateDet)/LL State Machine Conditions (LLSMCon)/Disable Condition (DisblC)/Subsystem/Subsystem15 ==
  in1 : Inport
  Add : Sum
  Cast To Single : DataTypeConversion  OutDataTypeStr=uint8
  Memory : Memory  InheritSampleTime=on
  Saturation : Saturate  UpperLimit=1  LowerLimit=0
      settings: AttributesFormatString="Min = %<LowerLimit>  Max = %<UpperLimit>"
  Out1 : Outport
  wires:
  Cast To Single/1 -> Add/1
  in1/1 -> Cast To Single/1
  Memory/1 -> Saturation/1
  Add/1 -> Memory/1
  Saturation/1 -> Add/2, Out1/1

== system LKAS_AutoSave_20220216_1647/LKAS/LL/LLOn/LL State Determination (LLStateDet)/LL State Machine Conditions (LLSMCon)/Disable Condition (DisblC)/Subsystem/Subsystem16 ==
  in1 : Inport
  Add : Sum
  Cast To Single : DataTypeConversion  OutDataTypeStr=uint8
  Memory : Memory  InheritSampleTime=on
  Saturation : Saturate  UpperLimit=1  LowerLimit=0
      settings: AttributesFormatString="Min = %<LowerLimit>  Max = %<UpperLimit>"
  Out1 : Outport
  wires:
  Cast To Single/1 -> Add/1
  in1/1 -> Cast To Single/1
  Memory/1 -> Saturation/1
  Add/1 -> Memory/1
  Saturation/1 -> Add/2, Out1/1

== system LKAS_AutoSave_20220216_1647/LKAS/LL/LLOn/LL State Determination (LLStateDet)/LL State Machine Conditions (LLSMCon)/Disable Condition (DisblC)/Subsystem/Subsystem17 ==
  in1 : Inport
  Add : Sum
  Cast To Single : DataTypeConversion  OutDataTypeStr=uint8
  Memory : Memory  InheritSampleTime=on
  Saturation : Saturate  UpperLimit=1  LowerLimit=0
      settings: AttributesFormatString="Min = %<LowerLimit>  Max = %<UpperLimit>"
  Out1 : Outport
  wires:
  Saturation/1 -> Out1/1, Add/2
  Add/1 -> Memory/1
  Memory/1 -> Saturation/1
  in1/1 -> Cast To Single/1
  Cast To Single/1 -> Add/1

== system LKAS_AutoSave_20220216_1647/LKAS/LL/LLOn/LL State Determination (LLStateDet)/LL State Machine Conditions (LLSMCon)/Disable Condition (DisblC)/Subsystem/Subsystem2 ==
  in1 : Inport
  Add : Sum
  Cast To Single : DataTypeConversion  OutDataTypeStr=uint8
  Memory : Memory  InheritSampleTime=on
  Saturation : Saturate  UpperLimit=1  LowerLimit=0
      settings: AttributesFormatString="Min = %<LowerLimit>  Max = %<UpperLimit>"
  Out1 : Outport
  wires:
  Saturation/1 -> Out1/1, Add/2
  Add/1 -> Memory/1
  Memory/1 -> Saturation/1
  in1/1 -> Cast To Single/1
  Cast To Single/1 -> Add/1

== system LKAS_AutoSave_20220216_1647/LKAS/LL/LLOn/LL State Determination (LLStateDet)/LL State Machine Conditions (LLSMCon)/Disable Condition (DisblC)/Subsystem/Subsystem3 ==
  in1 : Inport
  Add : Sum
  Cast To Single : DataTypeConversion  OutDataTypeStr=uint8
  Memory : Memory  InheritSampleTime=on
  Saturation : Saturate  UpperLimit=1  LowerLimit=0
      settings: AttributesFormatString="Min = %<LowerLimit>  Max = %<UpperLimit>"
  Out1 : Outport
  wires:
  Cast To Single/1 -> Add/1
  in1/1 -> Cast To Single/1
  Memory/1 -> Saturation/1
  Add/1 -> Memory/1
  Saturation/1 -> Add/2, Out1/1

== system LKAS_AutoSave_20220216_1647/LKAS/LL/LLOn/LL State Determination (LLStateDet)/LL State Machine Conditions (LLSMCon)/Disable Condition (DisblC)/Subsystem/Subsystem4 ==
  in1 : Inport
  Add : Sum
  Cast To Single : DataTypeConversion  OutDataTypeStr=uint8
  Memory : Memory  InheritSampleTime=on
  Saturation : Saturate  UpperLimit=1  LowerLimit=0
      settings: AttributesFormatString="Min = %<LowerLimit>  Max = %<UpperLimit>"
  Out1 : Outport
  wires:
  Saturation/1 -> Out1/1, Add/2
  Add/1 -> Memory/1
  Memory/1 -> Saturation/1
  in1/1 -> Cast To Single/1
  Cast To Single/1 -> Add/1

== system LKAS_AutoSave_20220216_1647/LKAS/LL/LLOn/LL State Determination (LLStateDet)/LL State Machine Conditions (LLSMCon)/Disable Condition (DisblC)/Subsystem/Subsystem5 ==
  in1 : Inport
  Add : Sum
  Cast To Single : DataTypeConversion  OutDataTypeStr=uint8
  Memory : Memory  InheritSampleTime=on
  Saturation : Saturate  UpperLimit=1  LowerLimit=0
      settings: AttributesFormatString="Min = %<LowerLimit>  Max = %<UpperLimit>"
  Out1 : Outport
  wires:
  Cast To Single/1 -> Add/1
  in1/1 -> Cast To Single/1
  Memory/1 -> Saturation/1
  Add/1 -> Memory/1
  Saturation/1 -> Add/2, Out1/1

== system LKAS_AutoSave_20220216_1647/LKAS/LL/LLOn/LL State Determination (LLStateDet)/LL State Machine Conditions (LLSMCon)/Disable Condition (DisblC)/Subsystem/Subsystem6 ==
  in1 : Inport
  Add : Sum
  Cast To Single : DataTypeConversion  OutDataTypeStr=uint8
  Memory : Memory  InheritSampleTime=on
  Saturation : Saturate  UpperLimit=1  LowerLimit=0
      settings: AttributesFormatString="Min = %<LowerLimit>  Max = %<UpperLimit>"
  Out1 : Outport
  wires:
  Cast To Single/1 -> Add/1
  in1/1 -> Cast To Single/1
  Memory/1 -> Saturation/1
  Add/1 -> Memory/1
  Saturation/1 -> Add/2, Out1/1

== system LKAS_AutoSave_20220216_1647/LKAS/LL/LLOn/LL State Determination (LLStateDet)/LL State Machine Conditions (LLSMCon)/Disable Condition (DisblC)/Subsystem/Subsystem7 ==
  in1 : Inport
  Add : Sum
  Cast To Single : DataTypeConversion  OutDataTypeStr=uint8
  Memory : Memory  InheritSampleTime=on
  Saturation : Saturate  UpperLimit=1  LowerLimit=0
      settings: AttributesFormatString="Min = %<LowerLimit>  Max = %<UpperLimit>"
  Out1 : Outport
  wires:
  Saturation/1 -> Out1/1, Add/2
  Add/1 -> Memory/1
  Memory/1 -> Saturation/1
  in1/1 -> Cast To Single/1
  Cast To Single/1 -> Add/1

== system LKAS_AutoSave_20220216_1647/LKAS/LL/LLOn/LL State Determination (LLStateDet)/LL State Machine Conditions (LLSMCon)/Disable Condition (DisblC)/Subsystem/Subsystem8 ==
  in1 : Inport
  Add : Sum
  Cast To Single : DataTypeConversion  OutDataTypeStr=uint8
  Memory : Memory  InheritSampleTime=on
  Saturation : Saturate  UpperLimit=1  LowerLimit=0
      settings: AttributesFormatString="Min = %<LowerLimit>  Max = %<UpperLimit>"
  Out1 : Outport
  wires:
  Saturation/1 -> Out1/1, Add/2
  Add/1 -> Memory/1
  Memory/1 -> Saturation/1
  in1/1 -> Cast To Single/1
  Cast To Single/1 -> Add/1

== system LKAS_AutoSave_20220216_1647/LKAS/LL/LLOn/LL State Determination (LLStateDet)/LL State Machine Conditions (LLSMCon)/Disable Condition (DisblC)/Subsystem/Subsystem9 ==
  in1 : Inport
  Add : Sum
  Cast To Single : DataTypeConversion  OutDataTypeStr=uint8
  Memory : Memory  InheritSampleTime=on
  Saturation : Saturate  UpperLimit=1  LowerLimit=0
      settings: AttributesFormatString="Min = %<LowerLimit>  Max = %<UpperLimit>"
  Out1 : Outport
  wires:
  Cast To Single/1 -> Add/1
  in1/1 -> Cast To Single/1
  Memory/1 -> Saturation/1
  Add/1 -> Memory/1
  Saturation/1 -> Add/2, Out1/1

== system LKAS_AutoSave_20220216_1647/LKAS/LL/LLOn/LL State Determination (LLStateDet)/LL State Machine Conditions (LLSMCon)/Disable Condition (DisblC)/Vehicle State Condition (VehStateC)/Emergency Light Enable Condition (EmgcyLghtEC) ==
  EmgcyLghtEC_bsStLampState : Inport
  EmgcyLghtEC_SingleLane_Disable_Swt : Inport  Port=2
  Add : Sum
  Bus Selector : BusSelector  OutputSignals=BCM_Double_Light,BCM_Left_Light,BCM_Right_Light
  Compare To Constant : simulink/Logic and Bit Operations/Compare To Constant  relop=>  const=1  OutDataTypeStr=boolean
  Compare To Constant1 : simulink/Logic and Bit Operations/Compare To Constant  relop=>=  const=3  OutDataTypeStr=boolean
  Constant : Constant  Value=3  OutDataTypeStr=single
  Constant1 : Constant  Value=-1  OutDataTypeStr=single
  Logical Operator : Logic  Operator=NOT  AllPortsSameDT=off  OutDataTypeStr=boolean
  Logical Operator1 : Logic  Operator=OR  Inputs=3  AllPortsSameDT=off  OutDataTypeStr=boolean
  Logical Operator2 : Logic  AllPortsSameDT=off  OutDataTypeStr=boolean
  Logical Operator3 : Logic  AllPortsSameDT=off  OutDataTypeStr=boolean
  Memory : Memory  InheritSampleTime=on
  Saturation : Saturate  UpperLimit=200  LowerLimit=-1
      settings: AttributesFormatString="Min = %<LowerLimit>  Max = %<UpperLimit>"
  Switch : Switch  Criteria=u2 > Threshold
  EmgcyLghtEC_stEmgcyLghtECFlg : Outport
  wires:
  EmgcyLghtEC_bsStLampState/1 -> Bus Selector/1
  Bus Selector/1 -> Compare To Constant1/1  "<BCM_Double_Light>"
  Logical Operator1/1 -> Switch/2
  Constant/1 -> Switch/1
  Constant1/1 -> Switch/3
  Switch/1 -> Add/1
  Add/1 -> Saturation/1
  Saturation/1 -> Compare To Constant/1, Memory/1
  Memory/1 -> Add/2
  Compare To Constant/1 -> EmgcyLghtEC_stEmgcyLghtECFlg/1
  EmgcyLghtEC_SingleLane_Disable_Swt/1 -> Logical Operator/1
  Compare To Constant1/1 -> Logical Operator1/1
  Bus Selector/2 -> Logical Operator2/1  "<BCM_Left_Light>"
  Logical Operator2/1 -> Logical Operator1/2
  Logical Operator/1 -> Logical Operator2/2, Logical Operator3/2
  Bus Selector/3 -> Logical Operator3/1  "<BCM_Right_Light>"
  Logical Operator3/1 -> Logical Operator1/3

== system LKAS_AutoSave_20220216_1647/LKAS/LL/LLOn/LL State Determination (LLStateDet)/LL State Machine Conditions (LLSMCon)/Disable Condition (DisblC)/Vehicle State Condition (VehStateC)/Gear Disable Condition (GearDC) ==
  In1 : Inport
  Compare To Constant : simulink/Logic and Bit Operations/Compare To Constant  relop=~=  const=3  OutDataTypeStr=boolean
  GearDC_stGearDCFlg : Outport
  wires:
  In1/1 -> Compare To Constant/1
  Compare To Constant/1 -> GearDC_stGearDCFlg/1

== system LKAS_AutoSave_20220216_1647/LKAS/LL/LLOn/LL State Determination (LLStateDet)/LL State Machine Conditions (LLSMCon)/Disable Condition (DisblC)/Vehicle State Condition (VehStateC)/Vehicle Speed Disable Condition (VehSpdDC) ==
  VehSpdDC_stDACMode : Inport
  VehSpdDC_vVehSpd : Inport  Port=2
  VehSpdDC_vLDWVehSpdMax_C : Inport  Port=3
  VehSpdDC_vLKAVehSpdMax_C : Inport  Port=4
  VehSpdDC_vVehSpdMin_C : Inport  Port=5
  Interval Test Dynamic : simulink/Logic and Bit Operations/Interval Test Dynamic  IntervalClosedRight=off  IntervalClosedLeft=off  OutDataTypeStr=boolean
      settings: SourceProductName=Simulink  SourceProductBaseCode=SL
  Logical Operator : Logic  Operator=NOT  AllPortsSameDT=off  OutDataTypeStr=boolean
  Switch : Switch  Threshold=2
  VehSpdDC_stVehSpdDCFlg : Outport
  wires:
  Interval Test Dynamic/1 -> Logical Operator/1
  VehSpdDC_vVehSpd/1 -> Interval Test Dynamic/2
  VehSpdDC_vVehSpdMin_C/1 -> Interval Test Dynamic/3
  Logical Operator/1 -> VehSpdDC_stVehSpdDCFlg/1
  VehSpdDC_stDACMode/1 -> Switch/2
  VehSpdDC_vLKAVehSpdMax_C/1 -> Switch/1
  Switch/1 -> Interval Test Dynamic/1
  VehSpdDC_vLDWVehSpdMax_C/1 -> Switch/3

== system LKAS_AutoSave_20220216_1647/LKAS/LL/LLOn/LL State Determination (LLStateDet)/LL State Machine Conditions (LLSMCon)/Disable Condition (DisblC)/Vehicle State Condition (VehStateC)/Vehicle State Condition Synthesis (VehStateCSyn) ==
  VehStateCSyn_stVehSpdDCFlg : Inport
  VehStateCSyn_stEmgcyLghtDCFlg : Inport  Port=2
  VehStateCSyn_stGearDCFlg : Inport  Port=3
  Logical Operator3 : Logic  Operator=OR  Inputs=3  AllPortsSameDT=off  OutDataTypeStr=boolean
  VehStateCSyn_stVehStateCSyn : Outport
  wires:
  VehStateCSyn_stVehSpdDCFlg/1 -> Logical Operator3/1
  VehStateCSyn_stGearDCFlg/1 -> Logical Operator3/3
  Logical Operator3/1 -> VehStateCSyn_stVehStateCSyn/1
  VehStateCSyn_stEmgcyLghtDCFlg/1 -> Logical Operator3/2

== system LKAS_AutoSave_20220216_1647/LKAS/LL/LLOn/LL State Determination (LLStateDet)/LL State Machine Conditions (LLSMCon)/Enable Condition (EnaC)/Enable Condition Synthesis (EnaCSyn)/If Action Subsystem ==
  Action Port : ActionPort  InitializeStates=reset
      settings: AttributesFormatString=states = %<InitializeStates>
  Constant : Constant  OutDataTypeStr=boolean  SampleTime=-1
  Out : Outport
      settings: AttributesFormatString=%<OutputWhenDisabled> = %<InitialOutput>
  wires:
  Constant/1 -> Out/1

== system LKAS_AutoSave_20220216_1647/LKAS/LL/LLOn/LL State Determination (LLStateDet)/LL State Machine Conditions (LLSMCon)/Enable Condition (EnaC)/Enable Condition Synthesis (EnaCSyn)/If Action Subsystem2 ==
  Action Port : ActionPort  InitializeStates=reset
      settings: AttributesFormatString=states = %<InitializeStates>
  Constant : Constant  OutDataTypeStr=boolean  SampleTime=-1
  Out : Outport
      settings: AttributesFormatString=%<OutputWhenDisabled> = %<InitialOutput>
  wires:
  Constant/1 -> Out/1

== system LKAS_AutoSave_20220216_1647/LKAS/LL/LLOn/LL State Determination (LLStateDet)/LL State Machine Conditions (LLSMCon)/Enable Condition (EnaC)/Enable Condition Synthesis (EnaCSyn)/If Action Subsystem3 ==
  Action Port : ActionPort  InitializeStates=reset
      settings: AttributesFormatString=states = %<InitializeStates>
  Constant : Constant  Value=0  OutDataTypeStr=boolean
  Out : Outport
      settings: AttributesFormatString=%<OutputWhenDisabled> = %<InitialOutput>
  wires:
  Constant/1 -> Out/1

== system LKAS_AutoSave_20220216_1647/LKAS/LL/LLOn/LL State Determination (LLStateDet)/LL State Machine Conditions (LLSMCon)/Enable Condition (EnaC)/Enable Condition Synthesis (EnaCSyn)/If Action Subsystem4 ==
  Action Port : ActionPort  InitializeStates=reset
      settings: AttributesFormatString=states = %<InitializeStates>
  Constant : Constant  Value=0  OutDataTypeStr=boolean
  Out : Outport
      settings: AttributesFormatString=%<OutputWhenDisabled> = %<InitialOutput>
  wires:
  Constant/1 -> Out/1

== system LKAS_AutoSave_20220216_1647/LKAS/LL/LLOn/LL State Determination (LLStateDet)/LL State Machine Conditions (LLSMCon)/Enable Condition (EnaC)/LDW Own Condition (LDWOwnC)/LDW Own Condition Synthesis (LDWOwnCSyn) ==
  LDWOwnCSyn_stDACMode : Inport
  LDWOwnCSyn_stVehPosChk : Inport  Port=2
  Compare To Constant : simulink/Logic and Bit Operations/Compare To Constant  relop=>=  const=1  OutDataTypeStr=boolean
  Compare To Constant1 : simulink/Logic and Bit Operations/Compare To Constant  relop===  const=1  OutDataTypeStr=boolean
  Logical Operator : Logic  AllPortsSameDT=off  OutDataTypeStr=boolean
  LDWOwnCSyn_stLDWOwnCSyn : Outport
  wires:
  LDWOwnCSyn_stDACMode/1 -> Compare To Constant/1
  LDWOwnCSyn_stVehPosChk/1 -> Compare To Constant1/1
  Compare To Constant/1 -> Logical Operator/1
  Compare To Constant1/1 -> Logical Operator/2
  Logical Operator/1 -> LDWOwnCSyn_stLDWOwnCSyn/1
